simulink model "controlAerobi"  (R2017b)
settings: Solver=FixedStepDiscrete  StartTime=0.0  StopTime=inf  FixedStep=Ts  RelTol=1e-3
InitFcn:
  | load Navio2_bus;
  | Ts=0.0025;
StopFcn:
  | %save_system('controlAerobi.slx');
  | %run('D:\Eclipse_Workspaces\workspace_rasp\AutoPilot\contAerobi\UpdateFiles\CopyBuildFiles.m');
undefined symbols (not defined in the file or in its folder): DiscIntNeverNeededParam
libraries: simulink x36, sharedutil x1, sharedtransform x1, dspsigops x1
(part 2 of 4)

== system controlAerobi/Controllers/Quadrotor_Controllers/Geometric_controller/attitude_tracking ==
  R_d_tracking : Inport
  DataSensor : Inport  Port=2
  ControlGains : Inport  Port=3
  ControlModes : Inport  Port=4
  Bus Selector : BusSelector  OutputSignals=GeometricGains.UAVparameters.J,GeometricGains.Gains.k_R,GeometricGains.Gains.k_Omega,GeometricGains.Gains.k_I,GeometricGains.Gains.c2,GeometricGains.Gains.sat_R
  Bus Selector1 : BusSelector  OutputSignals=attitude_.AngularPosition.roll,attitude_.AngularPosition.pitch,attitude_.AngularPosition.yaw,attitude_.AngularRates.droll,attitude_.AngularRates.dpitch,attitude_.AngularRates.dyaw
  Gain : Gain  Gain=0
  Generate_attitude_refereces : Subsystem
  attitude_geometric_control : MATLAB Function  TreatAsAtomicUnit=on
  drift : Constant  Value=[0;0;0]
  U2 : Outport
  U3 : Outport  Port=2
  U4 : Outport  Port=3
  wires:
  ControlModes/1 -> Generate_attitude_refereces/1(ControlModes)
  Generate_attitude_refereces/1(R_d) -> attitude_geometric_control/7(R_d)
  Generate_attitude_refereces/3(dOmega_d) -> attitude_geometric_control/9(dOmega_d)
  Generate_attitude_refereces/2(Omega_d) -> attitude_geometric_control/8(Omega_d)
  ControlGains/1 -> Bus Selector/1
  Bus Selector1/5 -> attitude_geometric_control/5(dpitch)  "<dpitch>"
  Bus Selector1/2 -> attitude_geometric_control/2(pitch)  "<pitch>"
  DataSensor/1 -> Bus Selector1/1
  Bus Selector1/4 -> attitude_geometric_control/4(droll)  "<droll>"
  Bus Selector/2 -> attitude_geometric_control/12(k_R)  "<k_R>"
  Bus Selector1/6 -> attitude_geometric_control/6(dyaw)  "<dyaw>"
  Bus Selector1/1 -> attitude_geometric_control/1(roll)  "<roll>"
  attitude_geometric_control/3(U4) -> U4/1  "U4"
  Bus Selector/3 -> attitude_geometric_control/13(k_Omega)  "<k_Omega>"
  Bus Selector/1 -> attitude_geometric_control/11(J)  "<J>"
  attitude_geometric_control/2(U3) -> U3/1  "U3"
  attitude_geometric_control/1(U2) -> U2/1  "U2"
  R_d_tracking/1 -> Generate_attitude_refereces/2(R_d_tracking)
  drift/1 -> attitude_geometric_control/17(drift)
  Bus Selector1/3 -> Gain/1  "<yaw>"
  Gain/1 -> attitude_geometric_control/3(yaw)
  Bus Selector/6 -> attitude_geometric_control/16(sat)  "<sat_R>"
  Bus Selector/5 -> attitude_geometric_control/15(c2)  "<c2>"
  Bus Selector/4 -> attitude_geometric_control/14(k_I)  "<k_I>"
  Generate_attitude_refereces/4(reset) -> attitude_geometric_control/10(reset)

== system controlAerobi/Controllers/Quadrotor_Controllers/Geometric_controller/trajectory_tracking ==
  DataSensor : Inport
  ControlGains : Inport  Port=2
  ControlModes : Inport  Port=3
  Bus Selector : BusSelector  OutputSignals=attitude_.AngularPosition.roll,attitude_.AngularPosition.pitch,attitude_.AngularPosition.yaw,position_.Position.x,position_.Position.y,position_.Position.z,position_.Velocity.dx,position_.Velocity.dy,position_.Velocity.dz
  Bus Selector1 : BusSelector  OutputSignals=GeometricGains.Gains.k_x,GeometricGains.Gains.k_v,GeometricGains.Gains.k_i,GeometricGains.Gains.c1,GeometricGains.Gains.sat_P,GeometricGains.UAVparameters.Mass
  Generate_tracking_referecnces : Subsystem
  trajectory_tracking : MATLAB Function  TreatAsAtomicUnit=on
  f : Outport
  R_d_tracking : Outport  Port=2
  wires:
  trajectory_tracking/2(R_d) -> R_d_tracking/1
  trajectory_tracking/1(f) -> f/1
  Generate_tracking_referecnces/2(v_d) -> trajectory_tracking/11(v_d)
  Generate_tracking_referecnces/3(ddx_d) -> trajectory_tracking/12(ddx_d)
  Generate_tracking_referecnces/1(x_d) -> trajectory_tracking/10(x_d)
  DataSensor/1 -> Generate_tracking_referecnces/1(DataSensor), Bus Selector/1
  Bus Selector/5 -> trajectory_tracking/5(py)  "<y>"
  Bus Selector/8 -> trajectory_tracking/8(vy)  "<dy>"
  Bus Selector/7 -> trajectory_tracking/7(vx)  "<dx>"
  Bus Selector/9 -> trajectory_tracking/9(vz)  "<dz>"
  Bus Selector/4 -> trajectory_tracking/4(px)  "<x>"
  Bus Selector/6 -> trajectory_tracking/6(pz)  "<z>"
  Bus Selector/3 -> trajectory_tracking/3(yaw)  "<yaw>"
  Bus Selector/1 -> trajectory_tracking/1(roll)  "<roll>"
  Bus Selector/2 -> trajectory_tracking/2(pitch)  "<pitch>"
  Generate_tracking_referecnces/4(b1_d) -> trajectory_tracking/13(b1_d)
  ControlGains/1 -> Bus Selector1/1
  Bus Selector1/6 -> trajectory_tracking/21(m)  "<Mass>"
  Bus Selector1/2 -> trajectory_tracking/17(k_v)  "<k_v>"
  Bus Selector1/1 -> trajectory_tracking/16(k_x)  "<k_x>"
  ControlModes/1 -> Generate_tracking_referecnces/2(ControlModes)
  Generate_tracking_referecnces/5(T) -> trajectory_tracking/14(T)
  Bus Selector1/3 -> trajectory_tracking/18(k_i)  "<k_i>"
  Bus Selector1/4 -> trajectory_tracking/19(c1)  "<c1>"
  Bus Selector1/5 -> trajectory_tracking/20(sat)  "<sat_P>"
  Generate_tracking_referecnces/6(reset) -> trajectory_tracking/15(reset)

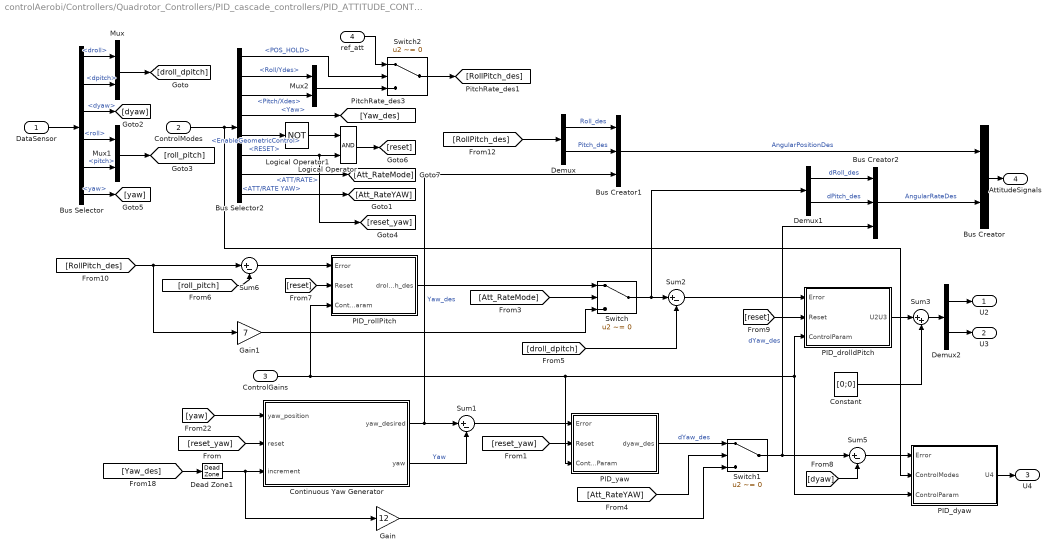
== system controlAerobi/Controllers/Quadrotor_Controllers/PID_cascade_controllers/PID_ATTITUDE_CONTROLLER ==
  DataSensor : Inport
  ControlModes : Inport  Port=2
  ControlGains : Inport  Port=3
  ref_att : Inport  Port=4
  Bus Creator : BusCreator  Inputs=2
  Bus Creator1 : BusCreator  Inputs=3
  Bus Creator2 : BusCreator  Inputs=3
  Bus Selector : BusSelector  OutputSignals=attitude_.AngularRates.droll,attitude_.AngularRates.dpitch,attitude_.AngularRates.dyaw,attitude_.AngularPosition.roll,attitude_.AngularPosition.pitch,attitude_.AngularPosition.yaw
  Bus Selector2 : BusSelector  OutputSignals=ModeControl.POS_HOLD,RemoteControl.Roll/Ydes,RemoteControl.Pitch/Xdes,RemoteControl.Yaw,ModeControl.EnableGeometricControl,ModeControl.RESET,ModeControl.ATT/RATE,ModeControl.ATT/RATE YAW
  Constant : Constant  Value=[0;0]
  Continuous Yaw Generator : MATLAB Function  TreatAsAtomicUnit=on
  Dead Zone1 : DeadZone  LowerValue=-0.025  UpperValue=0.025  SaturateOnIntegerOverflow=on
  Demux : Demux  Outputs=2
  Demux1 : Demux  Outputs=2
  Demux2 : Demux  Outputs=2
  Gain : Gain  Gain=12
  Gain1 : Gain  Gain=7
  Logical Operator : Logic  AllPortsSameDT=off  OutDataTypeStr=boolean
  Logical Operator1 : Logic  Operator=NOT  AllPortsSameDT=off  OutDataTypeStr=boolean
  Mux : Mux  Inputs=2
  Mux1 : Mux  Inputs=2
  Mux2 : Mux  Inputs=2
  PID_drolldPitch : Subsystem
  PID_dyaw : Subsystem
  PID_rollPitch : Subsystem
  PID_yaw : Subsystem
  Sum{1..2,5..6} (4 alike) : Sum  Inputs=|+-
  Sum3 : Sum  Inputs=|++
  Switch : Switch  Criteria=u2 ~= 0
  Switch1 : Switch  Criteria=u2 ~= 0
  Switch2 : Switch  Criteria=u2 ~= 0
  U2 : Outport
  U3 : Outport  Port=2
  U4 : Outport  Port=3
  AttitudeSignals : Outport  Port=4
  wires:
  Sum5/1 -> PID_dyaw/1(Error)
  [dyaw] -> Sum5/2
  [roll_pitch] -> Sum6/2
  [reset] -> PID_rollPitch/2(Reset)
  ControlModes/1 -> PID_dyaw/2(ControlModes), Bus Selector2/1
  PID_rollPitch/1(drolldpitch_des) -> Switch/1
  [reset_yaw] -> PID_yaw/2(Reset)
  Continuous Yaw Generator/1(yaw_desired) -> Sum1/1, Bus Creator1/3  "Yaw_des"
  [Yaw_des] -> Dead Zone1/1
  [reset_yaw] -> Continuous Yaw Generator/2(reset)
  [yaw] -> Continuous Yaw Generator/1(yaw_position)
  Continuous Yaw Generator/2(yaw) -> Sum1/2  "Yaw"
  [RollPitch_des] -> Sum6/1, Gain1/1
  Sum2/1 -> PID_drolldPitch/1(Error)
  [droll_dpitch] -> Sum2/2
  Switch/1 -> Demux1/1, Sum2/1
  Sum6/1 -> PID_rollPitch/1(Error)
  [Att_RateMode] -> Switch/2
  DataSensor/1 -> Bus Selector/1
  ControlGains/1 -> PID_rollPitch/3(ControlParam), PID_yaw/3(ControlParam), PID_dyaw/3(ControlParam), PID_drolldPitch/3(ControlParam)
  Bus Selector/3 -> [dyaw]  "<dyaw>"
  Bus Selector/1 -> Mux/1  "<droll>"
  Bus Selector/2 -> Mux/2  "<dpitch>"
  Bus Selector/4 -> Mux1/1  "<roll>"
  Bus Selector/5 -> Mux1/2  "<pitch>"
  Bus Selector/6 -> [yaw]  "<yaw>"
  Mux/1 -> [droll_dpitch]
  Mux1/1 -> [roll_pitch]
  Bus Selector2/2 -> Mux2/1  "<Roll/Ydes>"
  Bus Selector2/3 -> Mux2/2  "<Pitch/Xdes>"
  Bus Selector2/4 -> [Yaw_des]  "<Yaw>"
  Bus Selector2/7 -> [Att_RateMode]  "<ATT/RATE>"
  [reset] -> PID_drolldPitch/2(Reset)
  Demux2/1 -> U2/1
  Demux2/2 -> U3/1
  PID_dyaw/1(U4) -> U4/1
  Bus Creator/1 -> AttitudeSignals/1
  Sum1/1 -> PID_yaw/1(Error)
  PID_yaw/1(dyaw_des) -> Switch1/1  "dYaw_des"
  Switch1/1 -> Sum5/1, Bus Creator2/3  "dYaw_des"
  Bus Selector2/8 -> [Att_RateYAW]  "<ATT/RATE YAW>"
  [Att_RateYAW] -> Switch1/2
  Gain/1 -> Switch1/3
  Switch2/1 -> [RollPitch_des]
  Mux2/1 -> Switch2/3
  Bus Selector2/1 -> Switch2/2  "<POS_HOLD>"
  [RollPitch_des] -> Demux/1
  Demux/1 -> Bus Creator1/1  "Roll_des"
  Demux/2 -> Bus Creator1/2  "Pitch_des"
  Demux1/2 -> Bus Creator2/2  "dPitch_des"
  Demux1/1 -> Bus Creator2/1  "dRoll_des"
  Bus Creator2/1 -> Bus Creator/2  "AngularRateDes"
  Bus Creator1/1 -> Bus Creator/1  "AngularPositionDes"
  Gain1/1 -> Switch/3
  Dead Zone1/1 -> Gain/1, Continuous Yaw Generator/3(increment)
  Bus Selector2/5 -> Logical Operator1/1  "<EnableGeometricControl>"
  Bus Selector2/6 -> [reset_yaw], Logical Operator/2  "<RESET>"
  Logical Operator/1 -> [reset]
  Logical Operator1/1 -> Logical Operator/1
  Sum3/1 -> Demux2/1
  PID_drolldPitch/1(U2U3) -> Sum3/1
  Constant/1 -> Sum3/2
  ref_att/1 -> Switch2/1

== system controlAerobi/Controllers/Quadrotor_Controllers/PID_cascade_controllers/PID_POSITION_CONTROLLER ==
  DataSensor : Inport
  ControlModes : Inport  Port=2
  ControlGains : Inport  Port=3
  XY_controller : Subsystem
  Z_controller : Subsystem
  ref_att : Outport
  PositionSignals : Outport  Port=2
  AltitudeSignals : Outport  Port=3
  U1 : Outport  Port=4
  wires:
  Z_controller/2(U1) -> U1/1
  Z_controller/1(AltitudeSignals) -> AltitudeSignals/1
  XY_controller/1(PositionSignals) -> PositionSignals/1
  XY_controller/2(ref_att) -> ref_att/1
  ControlGains/1 -> XY_controller/1(ControlGains), Z_controller/1(ControlGains)
  DataSensor/1 -> XY_controller/2(DataSensor), Z_controller/2(DataSensor)
  ControlModes/1 -> Z_controller/3(ControlModes), XY_controller/3(ControlModes)

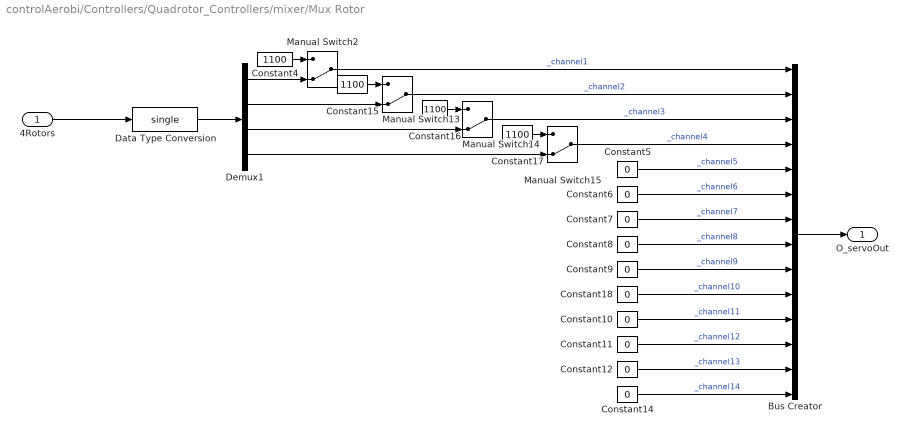
== system controlAerobi/Controllers/Quadrotor_Controllers/mixer/Mux Rotor ==
  4Rotors : Inport
  Bus Creator : BusCreator  Inputs=14
  Constant{5..12,14,18} (10 alike) : Constant  Value=0  OutDataTypeStr=single
  Constant{4,15..17} (4 alike) : Constant  Value=1100  OutDataTypeStr=uint16
  Data Type Conversion : DataTypeConversion  OutDataTypeStr=single
  Demux1 : Demux
  Manual Switch{2,13..15} (4 alike) : ManualSwitch  CurrentSetting=0
  O_servoOut : Outport  OutDataTypeStr=Bus: shm_RCou
  wires:
  Constant15/1 -> Manual Switch13/1
  Constant16/1 -> Manual Switch14/1
  Constant17/1 -> Manual Switch15/1
  Constant4/1 -> Manual Switch2/1
  Bus Creator/1 -> O_servoOut/1
  Manual Switch2/1 -> Bus Creator/1  "_channel1"
  Manual Switch13/1 -> Bus Creator/2  "_channel2"
  Manual Switch14/1 -> Bus Creator/3  "_channel3"
  Manual Switch15/1 -> Bus Creator/4  "_channel4"
  Constant5/1 -> Bus Creator/5  "_channel5"
  Constant6/1 -> Bus Creator/6  "_channel6"
  Constant7/1 -> Bus Creator/7  "_channel7"
  Constant8/1 -> Bus Creator/8  "_channel8"
  Constant9/1 -> Bus Creator/9  "_channel9"
  Constant18/1 -> Bus Creator/10  "_channel10"
  Constant10/1 -> Bus Creator/11  "_channel11"
  Constant11/1 -> Bus Creator/12  "_channel12"
  Constant12/1 -> Bus Creator/13  "_channel13"
  Constant14/1 -> Bus Creator/14  "_channel14"
  Data Type Conversion/1 -> Demux1/1
  Demux1/1 -> Manual Switch2/2
  Demux1/2 -> Manual Switch13/2
  Demux1/3 -> Manual Switch14/2
  Demux1/4 -> Manual Switch15/2
  4Rotors/1 -> Data Type Conversion/1

== system controlAerobi/Controllers/Quadrotor_Controllers/mixer/Subsystem ==
  CONTROL/MODE SIGNALS : Inport
  In2 : Inport  Port=2
  Bus Selector : BusSelector  OutputSignals=ModeControl.RESET
  Constant1 : Constant
  Constant2 : Constant  Value=0
  Product : Product
  Switch : Switch  Criteria=u2 ~= 0
  Out1 : Outport
  wires:
  Product/1 -> Out1/1
  In2/1 -> Product/2
  Constant1/1 -> Switch/1
  Switch/1 -> Product/1
  Bus Selector/1 -> Switch/2  "<RESET>"
  Constant2/1 -> Switch/3
  CONTROL/MODE SIGNALS/1 -> Bus Selector/1

== system controlAerobi/Controllers/Quadrotor_Controllers/mixer/saturation & Adapater signals ==
  thrust : Inport
  Roll : Inport  Port=2
  Pitch : Inport  Port=3
  Yaw : Inport  Port=4
  Constant1 : Constant  Value=inf
  Constant2 : Constant  Value=0
  Constant8 : Constant  Value=1227
  Gain{1,3,5,7} (4 alike) : Gain  Gain=6.5
  Sum1 : Sum  Inputs=|++
  ticks_Saturation Should Never saturate1 : simulink/Discontinuities/Saturation Dynamic  OutMin=[]  OutMax=[]  OutDataTypeStr=Inherit: Same as second input  OutDataType=fixdt(1, 16)  OutScaling=2^-10  DoSatur=off
  U1_out : Outport
  U2_out : Outport  Port=2
  U3_out : Outport  Port=3
  U4_out : Outport  Port=4
  wires:
  Constant2/1 -> ticks_Saturation Should Never saturate1/3
  Constant1/1 -> ticks_Saturation Should Never saturate1/1
  thrust/1 -> ticks_Saturation Should Never saturate1/2
  Pitch/1 -> Gain5/1
  Constant8/1 -> Sum1/2
  Sum1/1 -> U1_out/1
  Yaw/1 -> Gain7/1
  Gain1/1 -> Sum1/1
  ticks_Saturation Should Never saturate1/1 -> Gain1/1
  Gain3/1 -> U2_out/1
  Gain5/1 -> U3_out/1
  Gain7/1 -> U4_out/1
  Roll/1 -> Gain3/1

== system controlAerobi/Sensors/attitude/AttitudeEstimator/Acceleration ==
  accel : Inport
  Bus Creator1 : BusCreator  Inputs=3
  Demux1 : Demux  Outputs=3
  Accelerometer : Outport
  wires:
  Bus Creator1/1 -> Accelerometer/1  "Accelerometer"
  Demux1/1 -> Bus Creator1/1  "accelX"
  Demux1/2 -> Bus Creator1/2  "accelY"
  Demux1/3 -> Bus Creator1/3  "accelZ"
  accel/1 -> Demux1/1

== system controlAerobi/Sensors/attitude/AttitudeEstimator/AngularPosition ==
  attitude : Inport
  Bus Creator3 : BusCreator  Inputs=3
  Demux : Demux  Outputs=3
  attitude_ : Outport
  wires:
  Bus Creator3/1 -> attitude_/1
  Demux/2 -> Bus Creator3/2  "pitch"
  Demux/1 -> Bus Creator3/1  "roll"
  Demux/3 -> Bus Creator3/3  "yaw"
  attitude/1 -> Demux/1

== system controlAerobi/Sensors/attitude/AttitudeEstimator/AngularRates ==
  gyro : Inport
  Bus Creator : BusCreator  Inputs=3
  Demux1 : Demux  Outputs=3
  AngularRates : Outport
  wires:
  gyro/1 -> Demux1/1
  Bus Creator/1 -> AngularRates/1
  Demux1/1 -> Bus Creator/1  "droll"
  Demux1/2 -> Bus Creator/2  "dpitch"
  Demux1/3 -> Bus Creator/3  "dyaw"

== system controlAerobi/Sensors/attitude/AttitudeEstimator/DATA  ACQUISITION ==
  note: From PX4 (RPi+NAVIO)
  I_attitudePX4EKF2 : Inport  OutDataTypeStr=Bus: shm_attitudePX4EKF2
  "Demux UAV_att, UAV_att_rate" : Subsystem
  "PX4 + attitude " : Subsystem
  Zero-Order Hold1 : ZeroOrderHold  SampleTime=Ts
  vehicle_attitude : Outport
  vehicle_attitude_rate : Outport  Port=2
  wires:
  "Demux UAV_att, UAV_att_rate"/2(vehicle_attitude_rate) -> vehicle_attitude_rate/1
  Zero-Order Hold1/1 -> "Demux UAV_att, UAV_att_rate"/1(Att_topic)
  "PX4 + attitude "/1(attitude parameters) -> Zero-Order Hold1/1
  "Demux UAV_att, UAV_att_rate"/1(vehicle_attitude) -> vehicle_attitude/1
  I_attitudePX4EKF2/1 -> "PX4 + attitude "/1(I_attitudePX4EKF2)

== system controlAerobi/Sensors/attitude/AttitudeEstimator/calib accel lsm ==
  accel : Inport
  Add : Sum  Inputs=+-
  Bias accel : Constant  Value=[0.0758571454418519;0.0424696823519786;-0.321384803687075]
  M accel : Constant  Value=[0.102461992116242 -0.000598491957672618 0.000398970370700955;0 0.102027597979423 7.50526054392845e-05;0 0 0.101558166766067]
  Product : Product  Multiplication=Matrix(*)
  Rate Limiter1 : RateLimiter  RisingSlewLimit=10  FallingSlewLimit=-10  SampleTimeMode=inherited
  accel_ : Outport
  wires:
  M accel/1 -> Product/1
  Bias accel/1 -> Add/2
  Add/1 -> Product/2
  Product/1 -> Rate Limiter1/1
  accel/1 -> Add/1
  Rate Limiter1/1 -> accel_/1

== system controlAerobi/Sensors/attitude/AttitudeEstimator/calib gyro lsm ==
  gyro : Inport
  Add : Sum  Inputs=+-
  Bias gyro : Constant  Value=[0 0 0]
  M gyro : Constant  Value=[1 0 0;0 1 0;0 0 -1]
  MATLAB Function : MATLAB Function  TreatAsAtomicUnit=on
  Product : Product  Multiplication=Matrix(*)
  gyro_ : Outport
  wires:
  M gyro/1 -> Product/1
  gyro/1 -> Add/1
  Bias gyro/1 -> Add/2
  Add/1 -> MATLAB Function/1(g)
  Product/1 -> gyro_/1
  MATLAB Function/1(g_offset) -> Product/2

== system controlAerobi/Sensors/attitude/AttitudeEstimator/calib magnet lsm ==
  magnet : Inport
  Add : Sum  Inputs=+-
  Bias magnet : Constant  Value=[17.0874271396470;17.12515209882385;38.7277179953262]
  M magnet : Constant  Value=[0.0245576523410537 -0.00273259684033348 -0.00278802564696040;0 0.0254002563813822 -0.00118636240410959;0 0 -0.0239663665345273]
  Product : Product  Multiplication=Matrix(*)
  Rate Limiter1 : RateLimiter  RisingSlewLimit=10  FallingSlewLimit=-10  SampleTimeMode=inherited
  Security IsNaN2 : Subsystem
  magnet_ : Outport
  wires:
  Add/1 -> Product/2
  M magnet/1 -> Product/1
  Bias magnet/1 -> Add/2
  magnet/1 -> Add/1
  Rate Limiter1/1 -> Security IsNaN2/1(In1)
  Product/1 -> Rate Limiter1/1
  Security IsNaN2/1(Out1) -> magnet_/1

== system controlAerobi/Sensors/control_modes/ModeBlock/AdjustControlGain ==
  Channels : Inport
  Constant : Constant  Value=1512
  Constant1 : Constant  Value=800
  Data Type Conversion4 : DataTypeConversion  OutDataTypeStr=double
  Divide : Product  Inputs=*/
  Saturation : Saturate  UpperLimit=800  LowerLimit=-800
  Sum : Sum  Inputs=|+-
  man_auto switch channels 7 and 8 : Selector  InputPortWidth=10  IndexOptions=Index vector (dialog)  Indices=[7 6]  OutputSizes=1
  Gain : Outport
  wires:
  man_auto switch channels 7 and 8/1 -> Data Type Conversion4/1
  Channels/1 -> man_auto switch channels 7 and 8/1
  Data Type Conversion4/1 -> Sum/1
  Constant/1 -> Sum/2
  Sum/1 -> Saturation/1
  Saturation/1 -> Divide/1
  Divide/1 -> Gain/1
  Constant1/1 -> Divide/2

== system controlAerobi/Sensors/control_modes/Signals_to_references/Dead band_pitch ==
  in : Inport
  Abs : Abs
  Compare To Constant : simulink/Logic and Bit Operations/Compare To Constant  relop=<  const=0.01  OutDataTypeStr=uint8
  Constant : Constant  Value=0
  Switch : Switch  Criteria=u2 ~= 0
  out : Outport
  wires:
  in/1 -> Abs/1, Switch/3
  Abs/1 -> Compare To Constant/1
  Switch/1 -> out/1
  Constant/1 -> Switch/1
  Compare To Constant/1 -> Switch/2

== system controlAerobi/Sensors/control_modes/Signals_to_references/Dead band_roll ==
  in : Inport
  Abs : Abs
  Compare To Constant : simulink/Logic and Bit Operations/Compare To Constant  relop=<  const=0.01  OutDataTypeStr=uint8
  Constant : Constant  Value=0
  Switch : Switch  Criteria=u2 ~= 0
  out : Outport
  wires:
  Compare To Constant/1 -> Switch/2
  Constant/1 -> Switch/1
  Switch/1 -> out/1
  Abs/1 -> Compare To Constant/1
  in/1 -> Switch/3, Abs/1

== system controlAerobi/Sensors/control_modes/Signals_to_references/Dead band_yaw ==
  in : Inport
  Abs : Abs
  Compare To Constant : simulink/Logic and Bit Operations/Compare To Constant  relop=<  const=0.01  OutDataTypeStr=uint8
  Constant : Constant  Value=0
  Switch : Switch  Criteria=u2 ~= 0
  out : Outport
  wires:
  Compare To Constant/1 -> Switch/2
  Constant/1 -> Switch/1
  Switch/1 -> out/1
  Abs/1 -> Compare To Constant/1
  in/1 -> Switch/3, Abs/1

== system controlAerobi/Sensors/position/EKF_total_Station_Lidar/enu//ned ==
  I_totalStation : Inport  OutDataTypeStr=Bus: shm_totalStation
  Bus Selector2 : BusSelector  OutputSignals=_time,_y,_x
  Gain2 : Gain  OutDataTypeStr=double
  Gain3 : Gain  OutDataTypeStr=double
  NED/ENU : Constant
  Switch : Switch  Criteria=u2 ~= 0
  Switch1 : Switch  Criteria=u2 ~= 0
  timeTS : Outport
  x : Outport  Port=2
  y : Outport  Port=3
  wires:
  I_totalStation/1 -> Bus Selector2/1
  Bus Selector2/2 -> Gain3/1  "<_y>"
  Bus Selector2/3 -> Gain2/1  "<_x>"
  Bus Selector2/1 -> timeTS/1  "<_time>"
  Gain3/1 -> Switch1/3, Switch/1
  Gain2/1 -> Switch1/1, Switch/3
  Switch1/1 -> y/1
  Switch/1 -> x/1
  NED/ENU/1 -> Switch1/2, Switch/2

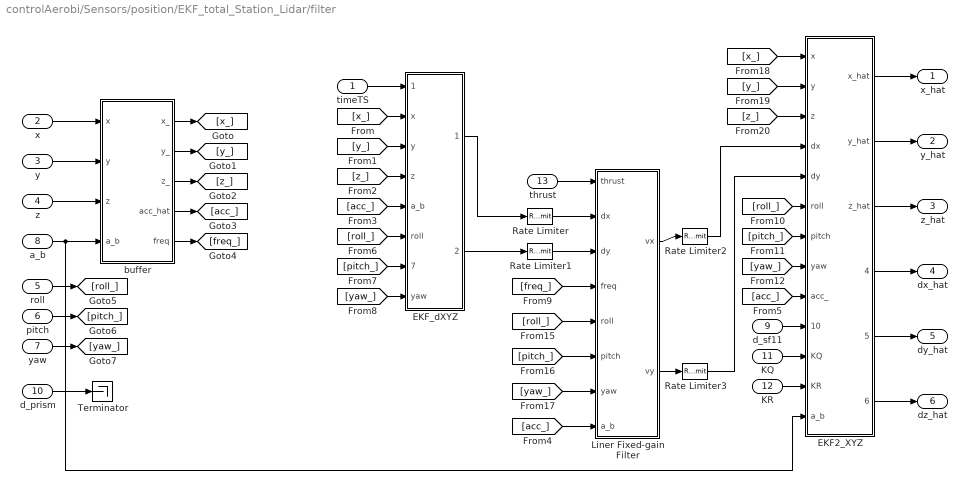
== system controlAerobi/Sensors/position/EKF_total_Station_Lidar/filter ==
  timeTS : Inport
  x : Inport  Port=2
  y : Inport  Port=3
  z : Inport  Port=4
  roll : Inport  Port=5
  pitch : Inport  Port=6
  yaw : Inport  Port=7
  a_b : Inport  Port=8
  d_sf11 : Inport  Port=9
  d_prism : Inport  Port=10
  KQ : Inport  Port=11
  KR : Inport  Port=12
  thrust : Inport  Port=13
  EKF2_XYZ : MATLAB Function  TreatAsAtomicUnit=on
  EKF_dXYZ : MATLAB Function  TreatAsAtomicUnit=on
  Liner Fixed-gain Filter : MATLAB Function  TreatAsAtomicUnit=on
  Rate Limiter{,1..3} (4 alike) : RateLimiter  RisingSlewLimit=5  FallingSlewLimit=-5  SampleTimeMode=inherited
  Terminator : Terminator
  buffer : MATLAB Function  TreatAsAtomicUnit=on
  x_hat : Outport
  y_hat : Outport  Port=2
  z_hat : Outport  Port=3
  dx_hat : Outport  Port=4
  dy_hat : Outport  Port=5
  dz_hat : Outport  Port=6
  wires:
  y/1 -> buffer/2(y)
  x/1 -> buffer/1(x)
  z/1 -> buffer/3(z)
  a_b/1 -> buffer/4(a_b), EKF2_XYZ/13(a_b)
  buffer/1(x_) -> [x_]
  buffer/2(y_) -> [y_]
  buffer/3(z_) -> [z_]
  [y_] -> EKF_dXYZ/3(y)
  [x_] -> EKF_dXYZ/2(x)
  [z_] -> EKF_dXYZ/4(z)
  buffer/4(acc_hat) -> [acc_]
  [acc_] -> EKF_dXYZ/5(a_b)
  [acc_] -> Liner Fixed-gain Filter/8(a_b)
  timeTS/1 -> EKF_dXYZ/1(timeTS)
  buffer/5(freq) -> [freq_]
  roll/1 -> [roll_]
  pitch/1 -> [pitch_]
  yaw/1 -> [yaw_]
  [freq_] -> Liner Fixed-gain Filter/4(freq)
  EKF_dXYZ/1(dx_hat) -> Rate Limiter/1
  EKF_dXYZ/2(dy_hat) -> Rate Limiter1/1
  thrust/1 -> Liner Fixed-gain Filter/1(thrust)
  Rate Limiter/1 -> Liner Fixed-gain Filter/2(dx)
  Rate Limiter1/1 -> Liner Fixed-gain Filter/3(dy)
  Liner Fixed-gain Filter/1(vx) -> Rate Limiter2/1
  Liner Fixed-gain Filter/2(vy) -> Rate Limiter3/1
  Rate Limiter2/1 -> EKF2_XYZ/4(dx)
  Rate Limiter3/1 -> EKF2_XYZ/5(dy)
  [roll_] -> EKF_dXYZ/6(roll)
  [pitch_] -> EKF_dXYZ/7(pitch)
  [yaw_] -> EKF_dXYZ/8(yaw)
  [roll_] -> EKF2_XYZ/6(roll)
  [pitch_] -> EKF2_XYZ/7(pitch)
  [yaw_] -> EKF2_XYZ/8(yaw)
  d_sf11/1 -> EKF2_XYZ/10(d_sf11)
  KQ/1 -> EKF2_XYZ/11(KQ)
  KR/1 -> EKF2_XYZ/12(KR)
  [roll_] -> Liner Fixed-gain Filter/5(roll)
  [pitch_] -> Liner Fixed-gain Filter/6(pitch)
  [yaw_] -> Liner Fixed-gain Filter/7(yaw)
  [x_] -> EKF2_XYZ/1(x)
  [y_] -> EKF2_XYZ/2(y)
  [z_] -> EKF2_XYZ/3(z)
  EKF2_XYZ/1(x_hat) -> x_hat/1
  EKF2_XYZ/2(y_hat) -> y_hat/1
  EKF2_XYZ/3(z_hat) -> z_hat/1
  EKF2_XYZ/4(dx_hat) -> dx_hat/1
  EKF2_XYZ/5(dy_hat) -> dy_hat/1
  EKF2_XYZ/6(dz_hat) -> dz_hat/1
  [acc_] -> EKF2_XYZ/9(acc_)
  d_prism/1 -> Terminator/1

== system controlAerobi/Sensors/position/EKF_total_Station_Lidar/routingData ==
  I_totalStation : Inport  OutDataTypeStr=Bus: shm_totalStation
  Bus Selector4 : BusSelector  OutputSignals=_x,_y,_z,_time
  Data{1..4} (4 alike) : DataTypeConversion  OutDataTypeStr=double
  Mux3 : Mux
  totalStation : Outport
  wires:
  I_totalStation/1 -> Bus Selector4/1
  Data4/1 -> Mux3/4
  Data1/1 -> Mux3/1
  Bus Selector4/4 -> Data4/1  "<_time>"
  Mux3/1 -> totalStation/1
  Bus Selector4/1 -> Data1/1  "<_x>"
  Data3/1 -> Mux3/3
  Bus Selector4/3 -> Data3/1  "<_z>"
  Bus Selector4/2 -> Data2/1  "<_y>"
  Data2/1 -> Mux3/2

== system controlAerobi/Sensors/position/GPS_px4/NED estimation ==
  I_localPositionPX4EKF2 : Inport  OutDataTypeStr=Bus: shm_localPositionPX4EKF2
  Bus Selector : BusSelector  OutputSignals=_x,_y,_z,_vx,_vy,_vz
  Demux : Demux  Outputs=2
  Mux : Mux  Inputs=6
  single2double : DataTypeConversion
  NED position : Outport
  NED speed : Outport  Port=2
  wires:
  single2double/1 -> Demux/1
  Demux/1 -> NED position/1
  Demux/2 -> NED speed/1
  I_localPositionPX4EKF2/1 -> Bus Selector/1
  Bus Selector/1 -> Mux/1  "<_x>"
  Bus Selector/2 -> Mux/2  "<_y>"
  Bus Selector/3 -> Mux/3  "<_z>"
  Bus Selector/4 -> Mux/4  "<_vx>"
  Bus Selector/5 -> Mux/5  "<_vy>"
  Bus Selector/6 -> Mux/6  "<_vz>"
  Mux/1 -> single2double/1

== system controlAerobi/Controllers/Quadrotor_Controllers/Geometric_controller/attitude_tracking/Generate_attitude_refereces ==
  ControlModes : Inport
  R_d_tracking : Inport  Port=2
  Bus Selector : BusSelector  OutputSignals=RemoteControl.Roll/Ydes,RemoteControl.Pitch/Xdes,RemoteControl.Yaw,ModeControl.RESET
  Calculate_rotation_matrix_des : MATLAB Function  TreatAsAtomicUnit=on
  Gain : Gain
  Gain1 : Gain  Gain=0
  Gain2 : Gain
  Gain3 : Gain  Gain=1.5
  Gain4 : Gain  Gain=1.5
  MATLAB Function : MATLAB Function  TreatAsAtomicUnit=on
  Terminator : Terminator
  calculate_dOmega_d : MATLAB Function  TreatAsAtomicUnit=on
  R_d : Outport
  Omega_d : Outport  Port=2
  dOmega_d : Outport  Port=3
  reset : Outport  Port=4
  wires:
  ControlModes/1 -> Bus Selector/1
  Bus Selector/1 -> MATLAB Function/1(roll), Gain4/1  "<Roll/Ydes>"
  Bus Selector/2 -> Gain3/1, MATLAB Function/2(pitch)  "<Pitch/Xdes>"
  Bus Selector/3 -> Gain1/1, MATLAB Function/3(yaw)  "<Yaw>"
  Calculate_rotation_matrix_des/1(R_d) -> R_d/1
  MATLAB Function/1(Omega_d) -> Gain2/1
  Gain/1 -> dOmega_d/1
  Gain1/1 -> Calculate_rotation_matrix_des/3(yaw)
  calculate_dOmega_d/1(dOmega_d) -> Gain/1
  R_d_tracking/1 -> Terminator/1
  Gain2/1 -> calculate_dOmega_d/1(Omegad), Omega_d/1
  Gain3/1 -> Calculate_rotation_matrix_des/2(pitch)
  Gain4/1 -> Calculate_rotation_matrix_des/1(roll)
  Bus Selector/4 -> reset/1  "<RESET>"

== system controlAerobi/Controllers/Quadrotor_Controllers/Geometric_controller/trajectory_tracking/Generate_tracking_referecnces ==
  DataSensor : Inport
  ControlModes : Inport  Port=2
  Bus Selector : BusSelector  OutputSignals=ModeControl.RESET,ModeControl.ALTHOLD
  Calculate_position_des : Subsystem
  Gain : Gain  Gain=0.6
  Gain1 : Gain
  Gain2 : Gain
  Logical Operator : Logic  AllPortsSameDT=off  OutDataTypeStr=boolean
  Mux : Mux  Inputs=3
  Position _desired_from_PC : Subsystem
  Switch2 : Switch  Criteria=u2 ~= 0
  b1 : Constant  Value=[1;0;0]
  calculate_altitude_des : Subsystem
  calculate_ddx_d : MATLAB Function  TreatAsAtomicUnit=on
  calculate_v_d : MATLAB Function  TreatAsAtomicUnit=on
  x_d : Outport
  v_d : Outport  Port=2
  ddx_d : Outport  Port=3
  b1_d : Outport  Port=4
  T : Outport  Port=5
  reset : Outport  Port=6
  wires:
  DataSensor/1 -> calculate_altitude_des/1(DataSensor), Calculate_position_des/1(DataSensor)
  ControlModes/1 -> Bus Selector/1, calculate_altitude_des/2(ControlModes), Position _desired_from_PC/1(ControlModes), Calculate_position_des/2(ControlModes)
  calculate_altitude_des/1(z_des) -> Mux/3
  Calculate_position_des/1(x_des) -> Mux/1
  Calculate_position_des/2(y_des) -> Mux/2
  Position _desired_from_PC/1(x_d) -> Switch2/1
  Position _desired_from_PC/2(EnablePC) -> Switch2/2
  Mux/1 -> Switch2/3
  b1/1 -> b1_d/1
  Switch2/1 -> calculate_v_d/1(x_d), x_d/1
  calculate_v_d/1(v_d) -> Gain2/1, calculate_ddx_d/1(v_d)
  calculate_ddx_d/1(ddx_d) -> Gain1/1
  Gain1/1 -> ddx_d/1
  calculate_altitude_des/2(T) -> Gain/1
  Gain/1 -> T/1
  Gain2/1 -> v_d/1
  Bus Selector/1 -> Logical Operator/1  "<RESET>"
  Bus Selector/2 -> Logical Operator/2  "<ALTHOLD>"
  Logical Operator/1 -> reset/1

== system controlAerobi/Controllers/Quadrotor_Controllers/PID_cascade_controllers/PID_ATTITUDE_CONTROLLER/PID_drolldPitch ==
  Error : Inport
  Reset : Inport  Port=2
  ControlParam : Inport  Port=3
  Bus Selector : BusSelector  OutputSignals=PIDgains.ROLL/PITCHcontroller.P_rate,PIDgains.ROLL/PITCHcontroller.I_rate,PIDgains.ROLL/PITCHcontroller.D_rate,PIDgains.ROLL/PITCHcontroller.Sat+_rate,PIDgains.ROLL/PITCHcontroller.Sat-_rate
  Clamping circuit1 : Subsystem
  Constant : Constant  Value=0
  Constant1 : Constant  Value=0
  Discrete Derivative : simulink/Discrete/Discrete Derivative  gainval=1.0  ICPrevScaledInput=0.0  InputProcessing=Inherited  OutMin=[]  OutMax=[]  OutDataType=fixdt(1, 16)  OutScaling=2^-10  DoSatur=off
  Discrete-Time Integrator : DiscreteIntegrator  ExternalReset=rising  SampleTime=Ts  ICPrevOutput=DiscIntNeverNeededParam  ICPrevScaledInput=DiscIntNeverNeededParam
  Product : Product  RndMeth=Zero
  Product1 : Product  RndMeth=Zero
  Product2 : Product  RndMeth=Zero
  Saturation Dynamic : simulink/Discontinuities/Saturation Dynamic  OutMin=[]  OutMax=[]  OutDataTypeStr=Inherit: Same as second input  OutDataType=fixdt(1, 16)  OutScaling=2^-10  DoSatur=off
  Sum : Sum  Inputs=+++
  Switch : Switch  Criteria=u2 > Threshold
  Switch4 : Switch  Criteria=u2 ~= 0
  U2U3 : Outport
  wires:
  Constant/1 -> Switch/1
  Product1/1 -> Clamping circuit1/3(preIntegrator), Switch/3
  Clamping circuit1/1(Clamp) -> Switch/2
  Switch/1 -> Discrete-Time Integrator/1
  Saturation Dynamic/1 -> Clamping circuit1/2(postSat), U2U3/1
  Discrete-Time Integrator/1 -> Sum/2
  Reset/1 -> Discrete-Time Integrator/2, Switch4/2
  Sum/1 -> Clamping circuit1/1(preSat), Saturation Dynamic/2
  Product/1 -> Sum/1
  Product2/1 -> Discrete Derivative/1
  Discrete Derivative/1 -> Sum/3
  ControlParam/1 -> Bus Selector/1
  Bus Selector/1 -> Product/1  "<P_rate>"
  Bus Selector/2 -> Product1/1  "<I_rate>"
  Bus Selector/3 -> Product2/1  "<D_rate>"
  Bus Selector/4 -> Saturation Dynamic/1  "<Sat+_rate>"
  Bus Selector/5 -> Saturation Dynamic/3  "<Sat-_rate>"
  Constant1/1 -> Switch4/3
  Switch4/1 -> Product1/2, Product/2, Product2/2
  Error/1 -> Switch4/1

== system controlAerobi/Controllers/Quadrotor_Controllers/PID_cascade_controllers/PID_ATTITUDE_CONTROLLER/PID_dyaw ==
  Error : Inport
  ControlModes : Inport  Port=2
  ControlParam : Inport  Port=3
  Bus Selector : BusSelector  OutputSignals=PIDgains.YAWcontroller.P_rate,PIDgains.YAWcontroller.I_rate,PIDgains.YAWcontroller.D_rate,PIDgains.YAWcontroller.Sat+_rate,PIDgains.YAWcontroller.Sat-_rate
  Bus Selector1 : BusSelector  OutputSignals=RemoteControl.Thrust/Zdes,ModeControl.RESET
  Clamping circuit1 : Subsystem
  Constant : Constant  Value=0
  Constant1 : Constant  Value=0
  Constant2 : Constant  Value=10
  Discrete Derivative : simulink/Discrete/Discrete Derivative  gainval=1.0  ICPrevScaledInput=0.0  InputProcessing=Inherited  OutMin=[]  OutMax=[]  OutDataType=fixdt(1, 16)  OutScaling=2^-10  DoSatur=off
  Discrete-Time Integrator : DiscreteIntegrator  ExternalReset=rising  SampleTime=Ts  ICPrevOutput=DiscIntNeverNeededParam  ICPrevScaledInput=DiscIntNeverNeededParam
  Product : Product  RndMeth=Zero
  Product1 : Product  RndMeth=Zero
  Product2 : Product  RndMeth=Zero
  Relational Operator : RelationalOperator  Operator=<=  OutDataTypeStr=boolean  RndMeth=Simplest
  Saturation Dynamic : simulink/Discontinuities/Saturation Dynamic  OutMin=[]  OutMax=[]  OutDataTypeStr=Inherit: Same as second input  OutDataType=fixdt(1, 16)  OutScaling=2^-10  DoSatur=off
  Sum : Sum  Inputs=+++
  Switch : Switch  Criteria=u2 > Threshold
  Switch1 : Switch  Criteria=u2 ~= 0
  Switch4 : Switch  Criteria=u2 ~= 0
  U4 : Outport
  wires:
  Error/1 -> Switch4/1
  Switch4/1 -> Product/2, Product2/2, Product1/2
  Constant1/1 -> Switch4/3
  Bus Selector/5 -> Saturation Dynamic/3  "<Sat-_rate>"
  Bus Selector/4 -> Saturation Dynamic/1  "<Sat+_rate>"
  Bus Selector/3 -> Product2/1  "<D_rate>"
  Bus Selector/2 -> Product1/1  "<I_rate>"
  Bus Selector/1 -> Product/1  "<P_rate>"
  ControlParam/1 -> Bus Selector/1
  Discrete Derivative/1 -> Sum/3
  Product2/1 -> Discrete Derivative/1
  Product/1 -> Sum/1
  Sum/1 -> Clamping circuit1/1(preSat), Saturation Dynamic/2
  Discrete-Time Integrator/1 -> Sum/2
  Saturation Dynamic/1 -> U4/1, Clamping circuit1/2(postSat)
  Switch/1 -> Discrete-Time Integrator/1
  Clamping circuit1/1(Clamp) -> Switch/2
  Constant/1 -> Switch1/1, Switch/1
  ControlModes/1 -> Bus Selector1/1
  Bus Selector1/2 -> Switch4/2, Discrete-Time Integrator/2  "<RESET>"
  Switch1/1 -> Clamping circuit1/3(preIntegrator), Switch/3
  Bus Selector1/1 -> Relational Operator/1  "<Thrust/Zdes>"
  Constant2/1 -> Relational Operator/2
  Relational Operator/1 -> Switch1/2
  Product1/1 -> Switch1/3

== system controlAerobi/Controllers/Quadrotor_Controllers/PID_cascade_controllers/PID_ATTITUDE_CONTROLLER/PID_rollPitch ==
  Error : Inport
  Reset : Inport  Port=2
  ControlParam : Inport  Port=3
  Bus Selector : BusSelector  OutputSignals=PIDgains.ROLL/PITCHcontroller.P_pos,PIDgains.ROLL/PITCHcontroller.I_pos,PIDgains.ROLL/PITCHcontroller.D_pos,PIDgains.ROLL/PITCHcontroller.Sat+_pos,PIDgains.ROLL/PITCHcontroller.Sat-_pos
  Clamping circuit1 : Subsystem
  Constant : Constant  Value=0
  Constant1 : Constant  Value=0
  Discrete Derivative : simulink/Discrete/Discrete Derivative  gainval=1.0  ICPrevScaledInput=0.0  InputProcessing=Inherited  OutMin=[]  OutMax=[]  OutDataType=fixdt(1, 16)  OutScaling=2^-10  DoSatur=off
  Discrete-Time Integrator : DiscreteIntegrator  ExternalReset=rising  SampleTime=Ts  ICPrevOutput=DiscIntNeverNeededParam  ICPrevScaledInput=DiscIntNeverNeededParam
  Product : Product  RndMeth=Zero
  Product1 : Product  RndMeth=Zero
  Product2 : Product  RndMeth=Zero
  Saturation Dynamic : simulink/Discontinuities/Saturation Dynamic  OutMin=[]  OutMax=[]  OutDataTypeStr=Inherit: Same as second input  OutDataType=fixdt(1, 16)  OutScaling=2^-10  DoSatur=off
  Sum : Sum  Inputs=+++
  Switch : Switch  Criteria=u2 > Threshold
  Switch4 : Switch  Criteria=u2 ~= 0
  drolldpitch_des : Outport
  wires:
  Error/1 -> Switch4/1
  Switch4/1 -> Product2/2, Product/2, Product1/2
  Constant1/1 -> Switch4/3
  Bus Selector/5 -> Saturation Dynamic/3  "<Sat-_pos>"
  Bus Selector/4 -> Saturation Dynamic/1  "<Sat+_pos>"
  Bus Selector/3 -> Product2/1  "<D_pos>"
  Bus Selector/2 -> Product1/1  "<I_pos>"
  Bus Selector/1 -> Product/1  "<P_pos>"
  ControlParam/1 -> Bus Selector/1
  Discrete Derivative/1 -> Sum/3
  Product2/1 -> Discrete Derivative/1
  Product/1 -> Sum/1
  Sum/1 -> Saturation Dynamic/2, Clamping circuit1/1(preSat)
  Reset/1 -> Switch4/2, Discrete-Time Integrator/2
  Discrete-Time Integrator/1 -> Sum/2
  Saturation Dynamic/1 -> drolldpitch_des/1, Clamping circuit1/2(postSat)
  Switch/1 -> Discrete-Time Integrator/1
  Clamping circuit1/1(Clamp) -> Switch/2
  Product1/1 -> Switch/3, Clamping circuit1/3(preIntegrator)
  Constant/1 -> Switch/1

== system controlAerobi/Controllers/Quadrotor_Controllers/PID_cascade_controllers/PID_ATTITUDE_CONTROLLER/PID_yaw ==
  Error : Inport
  Reset : Inport  Port=2
  ControlParam : Inport  Port=3
  Bus Selector : BusSelector  OutputSignals=PIDgains.YAWcontroller.P_pos,PIDgains.YAWcontroller.I_pos,PIDgains.YAWcontroller.D_pos,PIDgains.YAWcontroller.Sat+_pos,PIDgains.YAWcontroller.Sat-_pos
  Clamping circuit1 : Subsystem
  Constant : Constant  Value=0
  Constant1 : Constant  Value=0
  Discrete Derivative : simulink/Discrete/Discrete Derivative  gainval=1.0  ICPrevScaledInput=0.0  InputProcessing=Inherited  OutMin=[]  OutMax=[]  OutDataType=fixdt(1, 16)  OutScaling=2^-10  DoSatur=off
  Discrete-Time Integrator : DiscreteIntegrator  ExternalReset=rising  SampleTime=Ts  ICPrevOutput=DiscIntNeverNeededParam  ICPrevScaledInput=DiscIntNeverNeededParam
  Product : Product  RndMeth=Zero
  Product1 : Product  RndMeth=Zero
  Product2 : Product  RndMeth=Zero
  Saturation Dynamic : simulink/Discontinuities/Saturation Dynamic  OutMin=[]  OutMax=[]  OutDataTypeStr=Inherit: Same as second input  OutDataType=fixdt(1, 16)  OutScaling=2^-10  DoSatur=off
  Sum : Sum  Inputs=+++
  Switch : Switch  Criteria=u2 > Threshold
  Switch4 : Switch  Criteria=u2 ~= 0
  dyaw_des : Outport
  wires:
  Constant/1 -> Switch/1
  Product1/1 -> Clamping circuit1/3(preIntegrator), Switch/3
  Clamping circuit1/1(Clamp) -> Switch/2
  Switch/1 -> Discrete-Time Integrator/1
  Saturation Dynamic/1 -> Clamping circuit1/2(postSat), dyaw_des/1
  Discrete-Time Integrator/1 -> Sum/2
  Reset/1 -> Discrete-Time Integrator/2, Switch4/2
  Sum/1 -> Clamping circuit1/1(preSat), Saturation Dynamic/2
  Product/1 -> Sum/1
  Product2/1 -> Discrete Derivative/1
  Discrete Derivative/1 -> Sum/3
  ControlParam/1 -> Bus Selector/1
  Bus Selector/1 -> Product/1  "<P_pos>"
  Bus Selector/2 -> Product1/1  "<I_pos>"
  Bus Selector/3 -> Product2/1  "<D_pos>"
  Bus Selector/4 -> Saturation Dynamic/1  "<Sat+_pos>"
  Bus Selector/5 -> Saturation Dynamic/3  "<Sat-_pos>"
  Constant1/1 -> Switch4/3
  Switch4/1 -> Product1/2, Product/2, Product2/2
  Error/1 -> Switch4/1

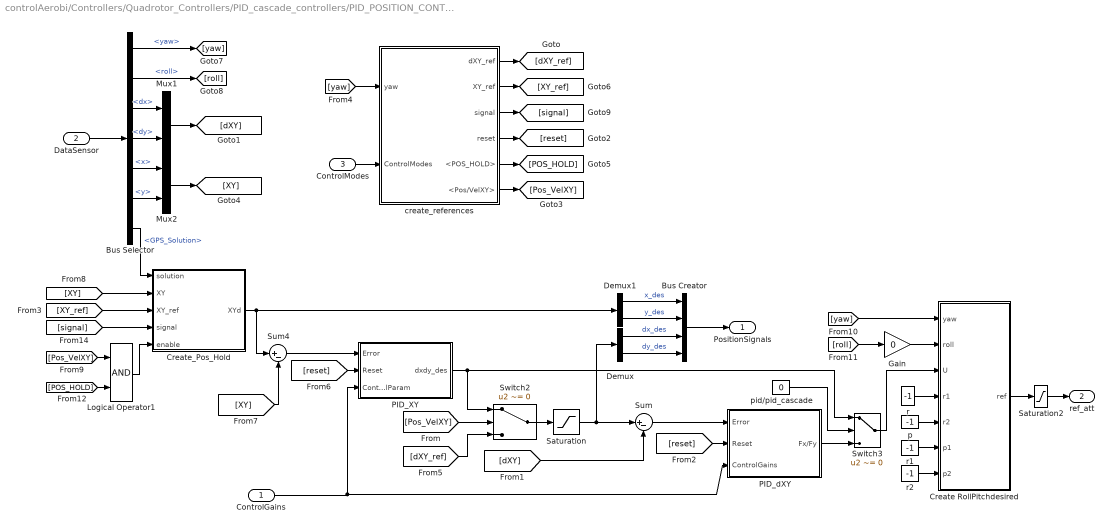
== system controlAerobi/Controllers/Quadrotor_Controllers/PID_cascade_controllers/PID_POSITION_CONTROLLER/XY_controller ==
  ControlGains : Inport
  DataSensor : Inport  Port=2
  ControlModes : Inport  Port=3
  Bus Creator : BusCreator  Inputs=4
  Bus Selector : BusSelector  OutputSignals=attitude_.AngularPosition.yaw,attitude_.AngularPosition.roll,position_.Velocity.dx,position_.Velocity.dy,position_.Position.x,position_.Position.y,position_.GPS_Solution
  Create RollPitchdesired : MATLAB Function  TreatAsAtomicUnit=on
  Create_Pos_Hold : MATLAB Function  TreatAsAtomicUnit=on
  Demux : Demux  Outputs=2
  Demux1 : Demux  Outputs=2
  Gain : Gain  Gain=0
  Logical Operator1 : Logic  AllPortsSameDT=off  OutDataTypeStr=boolean
  Mux1 : Mux  Inputs=2
  Mux2 : Mux  Inputs=2
  PID_XY : Subsystem
  PID_dXY : Subsystem
  Saturation : Saturate  UpperLimit=inf  LowerLimit=-inf
  Saturation2 : Saturate  UpperLimit=0.2  LowerLimit=-0.2
  Sum : Sum  Inputs=|+-
  Sum4 : Sum  Inputs=|+-
  Switch2 : Switch  Criteria=u2 ~= 0
  Switch3 : Switch  Criteria=u2 ~= 0
  create_references : Subsystem
  p : Constant  Value=-1
  pid/pid_cascade : Constant  Value=0
  r : Constant  Value=-1
  r1 : Constant  Value=-1
  r2 : Constant  Value=-1
  PositionSignals : Outport
  ref_att : Outport  Port=2
  wires:
  ControlGains/1 -> PID_XY/3(ControlParam), PID_dXY/3(ControlGains)
  DataSensor/1 -> Bus Selector/1
  Saturation/1 -> Demux/1, Sum/1
  Mux1/1 -> [dXY]
  [dXY] -> Sum/2
  [reset] -> PID_dXY/2(Reset)
  Bus Selector/3 -> Mux1/1  "<dx>"
  Bus Selector/4 -> Mux1/2  "<dy>"
  Bus Creator/1 -> PositionSignals/1
  Switch2/1 -> Saturation/1
  [Pos_VelXY] -> Switch2/2
  [dXY_ref] -> Switch2/3
  [reset] -> PID_XY/2(Reset)
  Bus Selector/5 -> Mux2/1  "<x>"
  Bus Selector/6 -> Mux2/2  "<y>"
  Mux2/1 -> [XY]
  [XY] -> Sum4/2
  Logical Operator1/1 -> Create_Pos_Hold/5(enable)
  [XY] -> Create_Pos_Hold/2(XY)
  [Pos_VelXY] -> Logical Operator1/1
  [POS_HOLD] -> Logical Operator1/2
  Sum4/1 -> PID_XY/1(Error)
  Sum/1 -> PID_dXY/1(Error)
  Demux/1 -> Bus Creator/3  "dx_des"
  Demux/2 -> Bus Creator/4  "dy_des"
  Demux1/1 -> Bus Creator/1  "x_des"
  Demux1/2 -> Bus Creator/2  "y_des"
  Create_Pos_Hold/1(XYd) -> Sum4/1, Demux1/1
  [XY_ref] -> Create_Pos_Hold/3(XY_ref)
  Create RollPitchdesired/1(ref) -> Saturation2/1
  Bus Selector/2 -> [roll]  "<roll>"
  Bus Selector/1 -> [yaw]  "<yaw>"
  [yaw] -> Create RollPitchdesired/1(yaw)
  [roll] -> Gain/1
  Saturation2/1 -> ref_att/1
  r/1 -> Create RollPitchdesired/4(r1)
  p/1 -> Create RollPitchdesired/5(r2)
  [signal] -> Create_Pos_Hold/4(signal)
  Bus Selector/7 -> Create_Pos_Hold/1(solution)  "<GPS_Solution>"
  Switch3/1 -> Create RollPitchdesired/3(U)
  PID_dXY/1(Fx/Fy) -> Switch3/3
  PID_XY/1(dxdy_des) -> Switch2/1, Switch3/1
  pid/pid_cascade/1 -> Switch3/2
  [yaw] -> create_references/1(yaw)
  ControlModes/1 -> create_references/2(ControlModes)
  create_references/1(dXY_ref) -> [dXY_ref]
  create_references/2(XY_ref) -> [XY_ref]
  create_references/3(signal) -> [signal]
  create_references/4(reset) -> [reset]
  create_references/5(<POS_HOLD>) -> [POS_HOLD]
  create_references/6(<Pos/VelXY>) -> [Pos_VelXY]
  Gain/1 -> Create RollPitchdesired/2(roll)
  r1/1 -> Create RollPitchdesired/6(p1)
  r2/1 -> Create RollPitchdesired/7(p2)

== system controlAerobi/Controllers/Quadrotor_Controllers/PID_cascade_controllers/PID_POSITION_CONTROLLER/Z_controller ==
  note: IF MODE==1 -> CONTROL  POS Z
      | IF MODE==0 -> CONTROL RATE Z
  ControlGains : Inport
  DataSensor : Inport  Port=2
  ControlModes : Inport  Port=3
  Altitude_PIDs : Subsystem
  Bus Creator : BusCreator  Inputs=2
  Bus Selector : BusSelector  OutputSignals=ModeControl.ALTHOLD,RemoteControl.Thrust/Zdes
  Switch1 : Switch  Criteria=u2 ~= 0
  calculate_altitude_des : Subsystem
  AltitudeSignals : Outport
  U1 : Outport  Port=2
  wires:
  Switch1/1 -> U1/1
  Altitude_PIDs/1(T) -> Switch1/1, Bus Creator/1  "Thrust"
  ControlGains/1 -> Altitude_PIDs/4(ControlGains)
  DataSensor/1 -> calculate_altitude_des/1(DataSensor), Altitude_PIDs/5(DataSensor)
  Altitude_PIDs/2(dZ_des) -> Bus Creator/2  "ZController"
  Bus Creator/1 -> AltitudeSignals/1
  calculate_altitude_des/2(Zdes) -> Altitude_PIDs/2(Zdes)
  calculate_altitude_des/3(dZdes) -> Altitude_PIDs/3(dZdes)
  calculate_altitude_des/1(T) -> Altitude_PIDs/1(TI)
  ControlModes/1 -> calculate_altitude_des/2(ControlModes), Altitude_PIDs/6(ControlModes), Bus Selector/1
  Bus Selector/1 -> Switch1/2  "<ALTHOLD>"
  Bus Selector/2 -> Switch1/3  "<Thrust/Zdes>"

== system controlAerobi/Sensors/attitude/AttitudeEstimator/DATA  ACQUISITION/Demux UAV_att, UAV_att_rate ==
  Att_topic : Inport
  Constant : Constant  Value=[0 0 0 1]
  Demux : Demux  Outputs=3
  Mux : Mux  Inputs=3
  Quaternion Norm : sharedutil/Quaternion Norm
      settings: SourceProductName=Aerospace Blockset  SourceProductBaseCode=AE
  Quaternions to Rotation Angles : sharedtransform/Quaternions to Rotation Angles  rotationOrder=ZYX
      settings: SourceProductBaseCode=AE
  Rotation Angles correction : Gain  Gain=[0 0 1;0 1 0;1 0 0]  Multiplication=Matrix(K*u)
  Switch : Switch  Criteria=u2 > Threshold
  Unwrap : dspsigops/Unwrap  tol=pi  InputProcessing=Columns as channels (frame based)  running=off
  u(1:3)[attitude rate] : Selector  InputPortWidth=7  IndexOptions=Index vector (dialog)  Indices=[1 2 3]  OutputSizes=1
  u(4:7)[quaternions] : Selector  InputPortWidth=7  IndexOptions=Index vector (dialog)  Indices=[4 5 6 7]  OutputSizes=1
  vehicle_attitude : Outport
  vehicle_attitude_rate : Outport  Port=2
  wires:
  Quaternions to Rotation Angles/1 -> Rotation Angles correction/1
  Att_topic/1 -> u(1:3)[attitude rate]/1, u(4:7)[quaternions]/1
  u(1:3)[attitude rate]/1 -> vehicle_attitude_rate/1
  u(4:7)[quaternions]/1 -> Quaternion Norm/1, Switch/1
  Quaternion Norm/1 -> Switch/2
  Switch/1 -> Quaternions to Rotation Angles/1
  Constant/1 -> Switch/3
  Demux/3 -> Unwrap/1
  Unwrap/1 -> Mux/3
  Demux/2 -> Mux/2
  Demux/1 -> Mux/1
  Rotation Angles correction/1 -> Demux/1
  Mux/1 -> vehicle_attitude/1

== system controlAerobi/Sensors/attitude/AttitudeEstimator/DATA  ACQUISITION/PX4 + attitude  ==
  I_attitudePX4EKF2 : Inport  OutDataTypeStr=Bus: shm_attitudePX4EKF2
  Bus Selector : BusSelector  OutputSignals=_rollspeed,_pitchspeed,_yawspeed,_q
  Mux : Mux
  single2double : DataTypeConversion
  attitude parameters : Outport
  wires:
  I_attitudePX4EKF2/1 -> Bus Selector/1
  Bus Selector/1 -> Mux/1  "<_rollspeed>"
  Bus Selector/2 -> Mux/2  "<_pitchspeed>"
  Bus Selector/3 -> Mux/3  "<_yawspeed>"
  Bus Selector/4 -> Mux/4  "<_q>"
  Mux/1 -> single2double/1
  single2double/1 -> attitude parameters/1

== system controlAerobi/Sensors/attitude/AttitudeEstimator/calib magnet lsm/Security IsNaN2 ==
  In1 : Inport
  Constant : Constant  Value=[0.5879;0.0081;0.8091]
  Relational Operator : RelationalOperator  Operator=isNaN  OutDataTypeStr=boolean  RndMeth=Nearest
  Switch : Switch  Criteria=u2 ~= 0
  Out1 : Outport
  wires:
  Switch/1 -> Out1/1
  Constant/1 -> Switch/1
  In1/1 -> Relational Operator/1, Switch/3
  Relational Operator/1 -> Switch/2

== system controlAerobi/Controllers/Quadrotor_Controllers/Geometric_controller/trajectory_tracking/Generate_tracking_referecnces/Calculate_position_des ==
  DataSensor : Inport
  ControlModes : Inport  Port=2
  Bus Selector1 : BusSelector  OutputSignals=RemoteControl.Pitch/Xdes,RemoteControl.Roll/Ydes,ModeControl.RESET,ModeControl.POS_HOLD
  Bus Selector2 : BusSelector  OutputSignals=attitude_.AngularPosition.yaw
  Create dXY desired : MATLAB Function  TreatAsAtomicUnit=on
  Dead Zone : DeadZone  LowerValue=-0.05  UpperValue=0.05  SaturateOnIntegerOverflow=on
  Dead Zone1 : DeadZone  LowerValue=-0.05  UpperValue=0.05  SaturateOnIntegerOverflow=on
  Demux : Demux  Outputs=2
  Discrete-Time Integrator : DiscreteIntegrator  ExternalReset=rising  InitialConditionSetting=State (most efficient)  SampleTime=-1  ICPrevOutput=DiscIntNeverNeededParam  ICPrevScaledInput=DiscIntNeverNeededParam
  Gain : Gain  Gain=-3
  Gain1 : Gain  Gain=3
  Logical Operator : Logic  AllPortsSameDT=off  OutDataTypeStr=boolean
  Saturation1 : Saturate  UpperLimit=3  LowerLimit=-3
  Switch1 : Switch  Criteria=u2 ~= 0
  zero : Constant  Value=0
  x_des : Outport
  y_des : Outport  Port=2
  wires:
  Saturation1/1 -> Switch1/1
  Dead Zone1/1 -> Gain1/1
  Logical Operator/1 -> Switch1/2, Discrete-Time Integrator/2
  Gain/1 -> Create dXY desired/2(chan2)
  Bus Selector1/2 -> Dead Zone1/1  "<Roll/Ydes>"
  Bus Selector1/3 -> Logical Operator/1  "<RESET>"
  zero/1 -> Switch1/3
  Gain1/1 -> Create dXY desired/3(chan3)
  Switch1/1 -> Discrete-Time Integrator/1
  Bus Selector1/4 -> Logical Operator/2  "<POS_HOLD>"
  Dead Zone/1 -> Gain/1
  Bus Selector1/1 -> Dead Zone/1  "<Pitch/Xdes>"
  Create dXY desired/1(dXY_d) -> Saturation1/1
  Bus Selector2/1 -> Create dXY desired/1(yaw)  "<yaw>"
  ControlModes/1 -> Bus Selector1/1
  DataSensor/1 -> Bus Selector2/1
  Discrete-Time Integrator/1 -> Demux/1
  Demux/1 -> x_des/1
  Demux/2 -> y_des/1

== system controlAerobi/Controllers/Quadrotor_Controllers/Geometric_controller/trajectory_tracking/Generate_tracking_referecnces/Position _desired_from_PC ==
  ControlModes : Inport
  Bus Selector1 : BusSelector  OutputSignals=PositionDesired.Xdes,PositionDesired.Ydes,PositionDesired.Zdes,ModeControl.EnablePC
  Mux : Mux  Inputs=3
  x_d : Outport
  EnablePC : Outport  Port=2
  wires:
  Bus Selector1/4 -> EnablePC/1  "<EnablePC>"
  ControlModes/1 -> Bus Selector1/1
  Bus Selector1/1 -> Mux/1  "<Xdes>"
  Mux/1 -> x_d/1
  Bus Selector1/2 -> Mux/2  "<Ydes>"
  Bus Selector1/3 -> Mux/3  "<Zdes>"

== system controlAerobi/Controllers/Quadrotor_Controllers/Geometric_controller/trajectory_tracking/Generate_tracking_referecnces/calculate_altitude_des ==
  DataSensor : Inport
  ControlModes : Inport  Port=2
  Bus Selector : BusSelector  OutputSignals=RemoteControl.Thrust/Zdes,ModeControl.ALTHOLD
  Bus Selector1 : BusSelector  OutputSignals=position_.Position.z
  Saturation : Saturate  UpperLimit=inf  LowerLimit=0
  Sum : Sum  Inputs=|+-
  Sum1 : Sum  Inputs=|++
  altitude_fcn : MATLAB Function  TreatAsAtomicUnit=on
  antiwind_up_dzdes : Subsystem
  antiwind_up_zdes : Subsystem
  med_thrust : Constant  Value=52.23
  z_des : Outport
  T : Outport  Port=2
  wires:
  ControlModes/1 -> Bus Selector/1
  DataSensor/1 -> Bus Selector1/1
  Bus Selector/2 -> antiwind_up_zdes/2(reset), altitude_fcn/2(althold)  "<ALTHOLD>"
  Bus Selector/1 -> altitude_fcn/3(thrust), Sum/1  "<Thrust/Zdes>"
  med_thrust/1 -> Sum/2
  Bus Selector1/1 -> altitude_fcn/1(z)  "<z>"
  altitude_fcn/1(zdes) -> Sum1/2
  altitude_fcn/2(thrust_ini) -> T/1
  antiwind_up_zdes/1(I) -> Sum1/1
  Sum1/1 -> Saturation/1
  antiwind_up_dzdes/1(I) -> antiwind_up_zdes/1(error)
  Sum/1 -> antiwind_up_dzdes/1(error)
  Saturation/1 -> z_des/1

== system controlAerobi/Controllers/Quadrotor_Controllers/PID_cascade_controllers/PID_ATTITUDE_CONTROLLER/PID_drolldPitch/Clamping circuit1 ==
  preSat : Inport
  postSat : Inport  Port=2
  preIntegrator : Inport  Port=3
  AND : Logic  DisableCoverage=on  OutDataTypeStr=boolean
  Abs : Abs
  Add : Sum  Inputs=+-
  Compare To Constant : simulink/Logic and Bit Operations/Compare To Constant  relop=>=  const=1e-10  OutDataTypeStr=boolean
  Equal : RelationalOperator  DisableCoverage=on  Operator===  OutDataTypeStr=boolean  RndMeth=Nearest  InputSameDT=on
  SignPreIntegrator : Signum  DisableCoverage=on
  SignPreSat : Signum  DisableCoverage=on
  Clamp : Outport
  wires:
  Abs/1 -> Compare To Constant/1
  Add/1 -> Abs/1
  postSat/1 -> Add/2
  preSat/1 -> Add/1, SignPreSat/1
  preIntegrator/1 -> SignPreIntegrator/1
  SignPreSat/1 -> Equal/1
  Compare To Constant/1 -> AND/1
  SignPreIntegrator/1 -> Equal/2
  Equal/1 -> AND/2
  AND/1 -> Clamp/1

== system controlAerobi/Controllers/Quadrotor_Controllers/PID_cascade_controllers/PID_ATTITUDE_CONTROLLER/PID_dyaw/Clamping circuit1 ==
  preSat : Inport
  postSat : Inport  Port=2
  preIntegrator : Inport  Port=3
  AND : Logic  DisableCoverage=on  OutDataTypeStr=boolean
  Abs : Abs
  Add : Sum  Inputs=+-
  Compare To Constant : simulink/Logic and Bit Operations/Compare To Constant  relop=>=  const=1e-10  OutDataTypeStr=boolean
  Equal : RelationalOperator  DisableCoverage=on  Operator===  OutDataTypeStr=boolean  RndMeth=Nearest  InputSameDT=on
  SignPreIntegrator : Signum  DisableCoverage=on
  SignPreSat : Signum  DisableCoverage=on
  Clamp : Outport
  wires:
  AND/1 -> Clamp/1
  Equal/1 -> AND/2
  SignPreIntegrator/1 -> Equal/2
  Compare To Constant/1 -> AND/1
  SignPreSat/1 -> Equal/1
  preIntegrator/1 -> SignPreIntegrator/1
  preSat/1 -> SignPreSat/1, Add/1
  postSat/1 -> Add/2
  Add/1 -> Abs/1
  Abs/1 -> Compare To Constant/1

== system controlAerobi/Controllers/Quadrotor_Controllers/PID_cascade_controllers/PID_ATTITUDE_CONTROLLER/PID_rollPitch/Clamping circuit1 ==
  preSat : Inport
  postSat : Inport  Port=2
  preIntegrator : Inport  Port=3
  AND : Logic  DisableCoverage=on  OutDataTypeStr=boolean
  Abs : Abs
  Add : Sum  Inputs=+-
  Compare To Constant : simulink/Logic and Bit Operations/Compare To Constant  relop=>=  const=1e-10  OutDataTypeStr=boolean
  Equal : RelationalOperator  DisableCoverage=on  Operator===  OutDataTypeStr=boolean  RndMeth=Nearest  InputSameDT=on
  SignPreIntegrator : Signum  DisableCoverage=on
  SignPreSat : Signum  DisableCoverage=on
  Clamp : Outport
  wires:
  AND/1 -> Clamp/1
  Equal/1 -> AND/2
  SignPreIntegrator/1 -> Equal/2
  Compare To Constant/1 -> AND/1
  SignPreSat/1 -> Equal/1
  preIntegrator/1 -> SignPreIntegrator/1
  preSat/1 -> SignPreSat/1, Add/1
  postSat/1 -> Add/2
  Add/1 -> Abs/1
  Abs/1 -> Compare To Constant/1
